simulink model "Copy_of_VTOLTiltrotor"  (R2024a)
settings: configuration reference "VTOLConfiguration" (kept outside this file)
undefined symbols (not defined in the file): airspeed, Battery, BCE12, BCE_Set_init, BMS_Controller_State, C, Cell10_P, Cell11_P, Cell12_P, Cell1_N, Cell1_P, Cell2_P, Cell3_P, Cell4_P, Cell5_P, Cell6_P, Cell7_P, Cell8_P, Cell9_P, Cell_Temperatures, Cell_Voltages, Charging_State, CityMission, control, controlParams, ControlSampleTime, CriticalTiltAngle, currentFactor, CV_Gain, ddx, ddy, ddz, Device_01, DiscIntNeverNeededParam, dx, dy, dz, Earth, env, F, F28379D_ADC_MaxCount, F28379D_ADC_Vmax, FixedWingMission, flightState, Foc_Ki_IxTcpu, Foc_Ki_S, Foc_Kp_I, Foc_Kp_S, fractalcoef, FSState, FWControlParams, HoverMission, I_cc, Ia_offset, Ib_offset, iniRoll, initPitch, iniYaw, IO334, IO334_DAC_Vmax ... (+55)
libraries: slrealtimeethercatlib x109, simulink x81, fl_lib x65, slpidlib x49, mcbcontrolslib x48, nesl_utility x43, speedgoatlib_hdlCoder_IO3xx x31, canmsglib x17, slrealtimeutilitieslib x13, mcbhdlplantlib x13, speedgoatlib_IO611 x12, dspstat3 x12
(part 9 of 20)

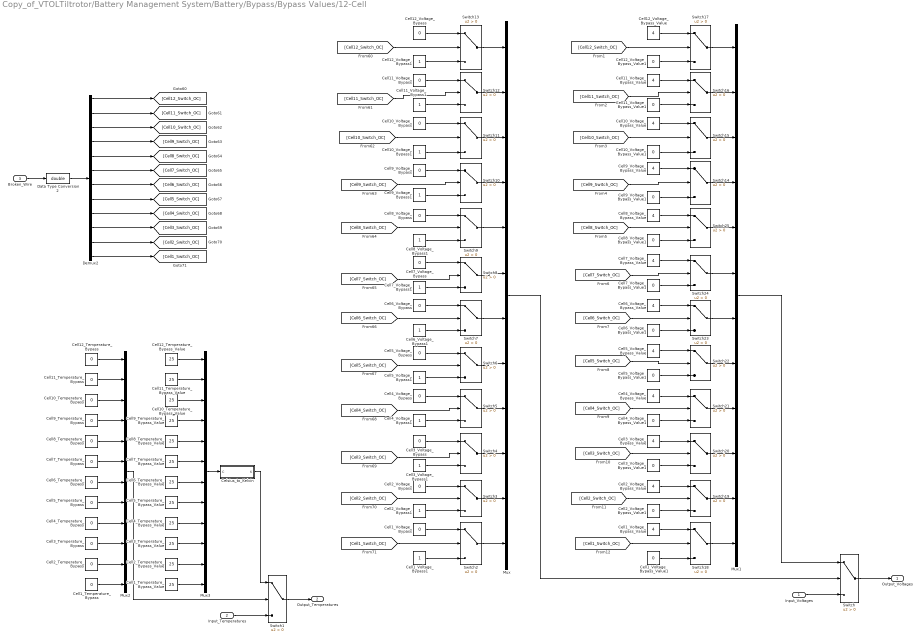
== system Copy_of_VTOLTiltrotor/Battery Management System/Battery/Bypass/Bypass Values/12-Cell ==
  Input_Voltages : Inport
  Input_Temperatures : Inport  Port=2
  Broken_Wire : Inport  Port=3
  Cell10_Temperature_Bypass : Constant  Value=0  SampleTime=-1
  Cell10_Temperature_Bypass_Value : Constant  Value=25  SampleTime=-1
  Cell10_Voltage_Bypass : Constant  Value=0  SampleTime=-1
  Cell10_Voltage_Bypass1 : Constant  SampleTime=-1
  Cell10_Voltage_Bypass_Value : Constant  Value=4  SampleTime=-1
  Cell10_Voltage_Bypass_Value1 : Constant  Value=0  SampleTime=-1
  Cell11_Temperature_Bypass : Constant  Value=0  SampleTime=-1
  Cell11_Temperature_Bypass_Value : Constant  Value=25  SampleTime=-1
  Cell11_Voltage_Bypass : Constant  Value=0  SampleTime=-1
  Cell11_Voltage_Bypass1 : Constant  SampleTime=-1
  Cell11_Voltage_Bypass_Value : Constant  Value=4  SampleTime=-1
  Cell11_Voltage_Bypass_Value1 : Constant  Value=0  SampleTime=-1
  Cell12_Temperature_Bypass : Constant  Value=0  SampleTime=-1
  Cell12_Temperature_Bypass_Value : Constant  Value=25  SampleTime=-1
  Cell12_Voltage_Bypass : Constant  Value=0  SampleTime=-1
  Cell12_Voltage_Bypass1 : Constant  SampleTime=-1
  Cell12_Voltage_Bypass_Value : Constant  Value=4  SampleTime=-1
  Cell12_Voltage_Bypass_Value1 : Constant  Value=0  SampleTime=-1
  Cell1_Temperature_Bypass : Constant  Value=0  SampleTime=-1
  Cell1_Temperature_Bypass_Value : Constant  Value=25  SampleTime=-1
  Cell1_Voltage_Bypass : Constant  Value=0  SampleTime=-1
  Cell1_Voltage_Bypass1 : Constant  SampleTime=-1
  Cell1_Voltage_Bypass_Value : Constant  Value=4  SampleTime=-1
  Cell1_Voltage_Bypass_Value1 : Constant  Value=0  SampleTime=-1
  Cell2_Temperature_Bypass : Constant  Value=0  SampleTime=-1
  Cell2_Temperature_Bypass_Value : Constant  Value=25  SampleTime=-1
  Cell2_Voltage_Bypass : Constant  Value=0  SampleTime=-1
  Cell2_Voltage_Bypass1 : Constant  SampleTime=-1
  Cell2_Voltage_Bypass_Value : Constant  Value=4  SampleTime=-1
  Cell2_Voltage_Bypass_Value1 : Constant  Value=0  SampleTime=-1
  Cell3_Temperature_Bypass : Constant  Value=0  SampleTime=-1
  Cell3_Temperature_Bypass_Value : Constant  Value=25  SampleTime=-1
  Cell3_Voltage_Bypass : Constant  Value=0  SampleTime=-1
  Cell3_Voltage_Bypass1 : Constant  SampleTime=-1
  Cell3_Voltage_Bypass_Value : Constant  Value=4  SampleTime=-1
  Cell3_Voltage_Bypass_Value1 : Constant  Value=0  SampleTime=-1
  Cell4_Temperature_Bypass : Constant  Value=0  SampleTime=-1
  Cell4_Temperature_Bypass_Value : Constant  Value=25  SampleTime=-1
  Cell4_Voltage_Bypass : Constant  Value=0  SampleTime=-1
  Cell4_Voltage_Bypass1 : Constant  SampleTime=-1
  Cell4_Voltage_Bypass_Value : Constant  Value=4  SampleTime=-1
  Cell4_Voltage_Bypass_Value1 : Constant  Value=0  SampleTime=-1
  Cell5_Temperature_Bypass : Constant  Value=0  SampleTime=-1
  Cell5_Temperature_Bypass_Value : Constant  Value=25  SampleTime=-1
  Cell5_Voltage_Bypass : Constant  Value=0  SampleTime=-1
  Cell5_Voltage_Bypass1 : Constant  SampleTime=-1
  Cell5_Voltage_Bypass_Value : Constant  Value=4  SampleTime=-1
  Cell5_Voltage_Bypass_Value1 : Constant  Value=0  SampleTime=-1
  Cell6_Temperature_Bypass : Constant  Value=0  SampleTime=-1
  Cell6_Temperature_Bypass_Value : Constant  Value=25  SampleTime=-1
  Cell6_Voltage_Bypass : Constant  Value=0  SampleTime=-1
  Cell6_Voltage_Bypass1 : Constant  SampleTime=-1
  Cell6_Voltage_Bypass_Value : Constant  Value=4  SampleTime=-1
  Cell6_Voltage_Bypass_Value1 : Constant  Value=0  SampleTime=-1
  Cell7_Temperature_Bypass : Constant  Value=0  SampleTime=-1
  Cell7_Temperature_Bypass_Value : Constant  Value=25  SampleTime=-1
  Cell7_Voltage_Bypass : Constant  Value=0  SampleTime=-1
  Cell7_Voltage_Bypass1 : Constant  SampleTime=-1
  Cell7_Voltage_Bypass_Value : Constant  Value=4  SampleTime=-1
  Cell7_Voltage_Bypass_Value1 : Constant  Value=0  SampleTime=-1
  Cell8_Temperature_Bypass : Constant  Value=0  SampleTime=-1
  Cell8_Temperature_Bypass_Value : Constant  Value=25  SampleTime=-1
  Cell8_Voltage_Bypass : Constant  Value=0  SampleTime=-1
  Cell8_Voltage_Bypass1 : Constant  SampleTime=-1
  Cell8_Voltage_Bypass_Value : Constant  Value=4  SampleTime=-1
  Cell8_Voltage_Bypass_Value1 : Constant  Value=0  SampleTime=-1
  Cell9_Temperature_Bypass : Constant  Value=0  SampleTime=-1
  Cell9_Temperature_Bypass_Value : Constant  Value=25  SampleTime=-1
  Cell9_Voltage_Bypass : Constant  Value=0  SampleTime=-1
  Cell9_Voltage_Bypass1 : Constant  SampleTime=-1
  Cell9_Voltage_Bypass_Value : Constant  Value=4  SampleTime=-1
  Cell9_Voltage_Bypass_Value1 : Constant  Value=0  SampleTime=-1
  Celsius_to_Kelvin : Subsystem
  Data Type Conversion2 : DataTypeConversion  OutDataTypeStr=double  SaturateOnIntegerOverflow=off  RndMeth=Floor
  Demux2 : Demux  Outputs=12
  Mux{,1..3} (4 alike) : Mux  Inputs=12
  Switch{,1..25} (26 alike) : Switch  Criteria=u2 > Threshold  SaturateOnIntegerOverflow=off  InputSameDT=off
  Output_Voltages : Outport
  Output_Temperatures : Outport  Port=2
  wires:
  Mux/1 -> Switch/2
  Switch/1 -> Output_Voltages/1
  Mux1/1 -> Switch/1
  Input_Voltages/1 -> Switch/3
  Cell11_Temperature_Bypass/1 -> Mux2/2
  Cell1_Temperature_Bypass/1 -> Mux2/12
  Cell5_Temperature_Bypass/1 -> Mux2/8
  Cell6_Temperature_Bypass/1 -> Mux2/7
  Cell10_Temperature_Bypass/1 -> Mux2/3
  Cell4_Temperature_Bypass/1 -> Mux2/9
  Cell2_Temperature_Bypass/1 -> Mux2/11
  Cell9_Temperature_Bypass/1 -> Mux2/4
  Cell8_Temperature_Bypass_Value/1 -> Mux3/5
  Cell10_Temperature_Bypass_Value/1 -> Mux3/3
  Mux3/1 -> Celsius_to_Kelvin/1(C)
  Cell12_Temperature_Bypass_Value/1 -> Mux3/1
  Cell1_Temperature_Bypass_Value/1 -> Mux3/12
  Cell11_Temperature_Bypass_Value/1 -> Mux3/2
  Cell8_Temperature_Bypass/1 -> Mux2/5
  Cell3_Temperature_Bypass_Value/1 -> Mux3/10
  Cell9_Temperature_Bypass_Value/1 -> Mux3/4
  Cell6_Temperature_Bypass_Value/1 -> Mux3/7
  Cell12_Temperature_Bypass/1 -> Mux2/1
  Cell5_Temperature_Bypass_Value/1 -> Mux3/8
  Cell2_Temperature_Bypass_Value/1 -> Mux3/11
  Cell7_Temperature_Bypass/1 -> Mux2/6
  Mux2/1 -> Switch1/2
  Celsius_to_Kelvin/1(K) -> Switch1/1
  Cell4_Temperature_Bypass_Value/1 -> Mux3/9
  Input_Temperatures/1 -> Switch1/3
  Cell3_Temperature_Bypass/1 -> Mux2/10
  Cell7_Temperature_Bypass_Value/1 -> Mux3/6
  Switch1/1 -> Output_Temperatures/1
  Switch2/1 -> Mux/12
  [Cell5_Switch_OC] -> Switch6/2
  [Cell1_Switch_OC] -> Switch2/2
  [Cell8_Switch_OC] -> Switch9/2
  [Cell6_Switch_OC] -> Switch7/2
  [Cell7_Switch_OC] -> Switch8/2
  [Cell10_Switch_OC] -> Switch11/2
  [Cell12_Switch_OC] -> Switch13/2
  [Cell3_Switch_OC] -> Switch4/2
  [Cell9_Switch_OC] -> Switch10/2
  [Cell4_Switch_OC] -> Switch5/2
  [Cell11_Switch_OC] -> Switch12/2
  [Cell2_Switch_OC] -> Switch3/2
  Switch3/1 -> Mux/11
  Switch13/1 -> Mux/1
  Switch12/1 -> Mux/2
  Switch11/1 -> Mux/3
  Switch10/1 -> Mux/4
  Switch9/1 -> Mux/5
  Switch8/1 -> Mux/6
  Switch7/1 -> Mux/7
  Switch6/1 -> Mux/8
  Switch5/1 -> Mux/9
  Switch4/1 -> Mux/10
  Cell1_Voltage_Bypass/1 -> Switch2/1
  Cell2_Voltage_Bypass/1 -> Switch3/1
  Cell12_Voltage_Bypass/1 -> Switch13/1
  Cell11_Voltage_Bypass/1 -> Switch12/1
  Cell10_Voltage_Bypass/1 -> Switch11/1
  Cell9_Voltage_Bypass/1 -> Switch10/1
  Cell8_Voltage_Bypass/1 -> Switch9/1
  Cell7_Voltage_Bypass/1 -> Switch8/1
  Cell6_Voltage_Bypass/1 -> Switch7/1
  Cell5_Voltage_Bypass/1 -> Switch6/1
  Cell4_Voltage_Bypass/1 -> Switch5/1
  Cell3_Voltage_Bypass/1 -> Switch4/1
  Cell1_Voltage_Bypass1/1 -> Switch2/3
  Cell2_Voltage_Bypass1/1 -> Switch3/3
  Cell3_Voltage_Bypass1/1 -> Switch4/3
  Cell4_Voltage_Bypass1/1 -> Switch5/3
  Cell5_Voltage_Bypass1/1 -> Switch6/3
  Cell6_Voltage_Bypass1/1 -> Switch7/3
  Cell7_Voltage_Bypass1/1 -> Switch8/3
  Cell8_Voltage_Bypass1/1 -> Switch9/3
  Cell9_Voltage_Bypass1/1 -> Switch10/3
  Cell10_Voltage_Bypass1/1 -> Switch11/3
  Cell11_Voltage_Bypass1/1 -> Switch12/3
  Cell12_Voltage_Bypass1/1 -> Switch13/3
  Switch17/1 -> Mux1/1
  Switch16/1 -> Mux1/2
  Switch18/1 -> Mux1/12
  Switch25/1 -> Mux1/5
  Switch20/1 -> Mux1/10
  Switch19/1 -> Mux1/11
  Switch15/1 -> Mux1/3
  Switch14/1 -> Mux1/4
  Switch24/1 -> Mux1/6
  Switch23/1 -> Mux1/7
  Switch22/1 -> Mux1/8
  Switch21/1 -> Mux1/9
  Cell12_Voltage_Bypass_Value/1 -> Switch17/1
  Cell11_Voltage_Bypass_Value/1 -> Switch16/1
  Cell10_Voltage_Bypass_Value/1 -> Switch15/1
  Cell9_Voltage_Bypass_Value/1 -> Switch14/1
  Cell8_Voltage_Bypass_Value/1 -> Switch25/1
  Cell6_Voltage_Bypass_Value/1 -> Switch23/1
  Cell5_Voltage_Bypass_Value/1 -> Switch22/1
  Cell4_Voltage_Bypass_Value/1 -> Switch21/1
  Cell3_Voltage_Bypass_Value/1 -> Switch20/1
  Cell2_Voltage_Bypass_Value/1 -> Switch19/1
  Cell1_Voltage_Bypass_Value/1 -> Switch18/1
  Cell7_Voltage_Bypass_Value/1 -> Switch24/1
  Cell12_Voltage_Bypass_Value1/1 -> Switch17/3
  Cell11_Voltage_Bypass_Value1/1 -> Switch16/3
  Cell10_Voltage_Bypass_Value1/1 -> Switch15/3
  Cell9_Voltage_Bypass_Value1/1 -> Switch14/3
  Cell8_Voltage_Bypass_Value1/1 -> Switch25/3
  Cell7_Voltage_Bypass_Value1/1 -> Switch24/3
  Cell6_Voltage_Bypass_Value1/1 -> Switch23/3
  Cell5_Voltage_Bypass_Value1/1 -> Switch22/3
  Cell4_Voltage_Bypass_Value1/1 -> Switch21/3
  Cell3_Voltage_Bypass_Value1/1 -> Switch20/3
  Cell2_Voltage_Bypass_Value1/1 -> Switch19/3
  Cell1_Voltage_Bypass_Value1/1 -> Switch18/3
  [Cell12_Switch_OC] -> Switch17/2
  [Cell10_Switch_OC] -> Switch15/2
  [Cell11_Switch_OC] -> Switch16/2
  [Cell9_Switch_OC] -> Switch14/2
  [Cell8_Switch_OC] -> Switch25/2
  [Cell7_Switch_OC] -> Switch24/2
  [Cell6_Switch_OC] -> Switch23/2
  [Cell5_Switch_OC] -> Switch22/2
  [Cell4_Switch_OC] -> Switch21/2
  [Cell3_Switch_OC] -> Switch20/2
  [Cell2_Switch_OC] -> Switch19/2
  [Cell1_Switch_OC] -> Switch18/2
  Demux2/6 -> [Cell7_Switch_OC]
  Demux2/12 -> [Cell1_Switch_OC]
  Broken_Wire/1 -> Data Type Conversion2/1
  Demux2/5 -> [Cell8_Switch_OC]
  Demux2/11 -> [Cell2_Switch_OC]
  Demux2/7 -> [Cell6_Switch_OC]
  Demux2/3 -> [Cell10_Switch_OC]
  Demux2/9 -> [Cell4_Switch_OC]
  Demux2/2 -> [Cell11_Switch_OC]
  Demux2/10 -> [Cell3_Switch_OC]
  Demux2/4 -> [Cell9_Switch_OC]
  Demux2/8 -> [Cell5_Switch_OC]
  Data Type Conversion2/1 -> Demux2/1
  Demux2/1 -> [Cell12_Switch_OC]

== system Copy_of_VTOLTiltrotor/Battery Management System/Battery/HW Interface/BCE - HIL/Battery Cell Emulator ==
  Sensor_Values_Sim : Inport
  "BCE Bus Packing " : Subsystem
  "BCE Read " : Subsystem  InitFcn=sg_bce.checkNumberOfBlocksGlobal(bdroot);  mask(bce_read){}
      settings: OpenFcn=sg_bce.openFcnRead;
      mask Help: eval('sg.utils.help.show(''io_main/refentry_bce_read'');')
      mask Display: disp('Speedgoat\nBMTS Read\nEtherCAT Bus: 0, Device: 1\nBCE12-0505');port_label('output',1,'Data');
  "BCE Setup " : Subsystem  LoadFcn=|  InitFcn=|  mask(bce_setup){}
      LoadFcn=|
      | sg_bce.createBusSignals;
      | sg_bce.setupEniCallback(gcb, bdroot);
      InitFcn=|
      | sg_bce.createBusSignals;
      | sg_bce.checkNumberOfBlocksGlobal(bdroot);
      | sg_bce.setupEniCallback(gcb, bdroot);
      settings: OpenFcn=sg_bce.openFcnSetup;
      mask Help: eval('sg.utils.help.show(''io_main/refentry_bce_setup'');')
      mask Display: disp('Speedgoat\nBattery Management Testing Systems\nEtherCAT Bus: 0\nSetup');
  "BCE Write " : Subsystem  InitFcn=sg_bce.checkNumberOfBlocksGlobal(bdroot);  mask(bce_write){}
      settings: OpenFcn=sg_bce.openFcnWrite;
      mask Help: eval('sg.utils.help.show(''io_main/refentry_bce_write'');')
      mask Display: disp('Speedgoat\nBMTS Write\nEtherCAT Bus: 0, Device: 1\nBCE12-0505');port_label('input',1,'Data');
  BCE_Init : Switch  Criteria=u2 > Threshold  SaturateOnIntegerOverflow=off  InputSameDT=off
  Bus Selector : BusSelector  OutputSignals=Cell_12.I,Cell_11.I,Cell_10.I,Cell_9.I,Cell_8.I,Cell_7.I,Cell_6.I,Cell_5.I,Cell_4.I,Cell_3.I,Cell_2.I,Cell_1.I
  Bus Selector1 : BusSelector  OutputSignals=Cell_Voltages
  Bus Selector2 : BusSelector  OutputSignals=Cell_12.V,Cell_11.V,Cell_10.V,Cell_9.V,Cell_8.V,Cell_7.V,Cell_6.V,Cell_5.V,Cell_4.V,Cell_3.V,Cell_2.V,Cell_1.V
  Constant : Constant  Value=[0,0,0,0,0,0,0,0,0,0,0,0]
  Data Type Conversion : DataTypeConversion  OutDataTypeStr=single  SaturateOnIntegerOverflow=off  RndMeth=Floor
  Data Type Conversion1 : DataTypeConversion  OutDataTypeStr=boolean  SaturateOnIntegerOverflow=off  RndMeth=Floor
  Data Type Conversion2 : DataTypeConversion  OutDataTypeStr=single  SaturateOnIntegerOverflow=off  RndMeth=Floor
  Demux : Demux  Outputs=12
  Enable : Constant
  Mux : Mux  Inputs=12
  Mux1 : Mux  Inputs=12
  No_current : Constant  Value=0
  Step : Step  Time=2
  Current_Values : Outport
  Cell_Voltages : Outport  Port=2
  wires:
  Sensor_Values_Sim/1 -> Bus Selector1/1
  BCE_Init/1 -> Demux/1
  "BCE Read "/1(Data) -> Bus Selector/1, Bus Selector2/1
  Constant/1 -> Data Type Conversion2/1
  Step/1 -> BCE_Init/2
  "BCE Bus Packing "/1(BCE Bus) -> "BCE Write "/1(Data)
  No_current/1 -> Data Type Conversion/1
  Data Type Conversion2/1 -> BCE_Init/3
  Bus Selector/1 -> Mux/1  "<I>"
  Bus Selector/2 -> Mux/2  "<I>"
  Bus Selector/3 -> Mux/3  "<I>"
  Bus Selector/4 -> Mux/4  "<I>"
  Bus Selector/5 -> Mux/5  "<I>"
  Bus Selector/6 -> Mux/6  "<I>"
  Bus Selector/7 -> Mux/7  "<I>"
  Bus Selector/8 -> Mux/8  "<I>"
  Bus Selector/9 -> Mux/9  "<I>"
  Bus Selector/10 -> Mux/10  "<I>"
  Bus Selector/11 -> Mux/11  "<I>"
  Bus Selector/12 -> Mux/12  "<I>"
  Mux/1 -> Current_Values/1
  Bus Selector2/1 -> Mux1/1  "<V>"
  Bus Selector2/2 -> Mux1/2  "<V>"
  Bus Selector2/3 -> Mux1/3  "<V>"
  Bus Selector2/4 -> Mux1/4  "<V>"
  Bus Selector2/5 -> Mux1/5  "<V>"
  Bus Selector2/6 -> Mux1/6  "<V>"
  Bus Selector2/7 -> Mux1/7  "<V>"
  Bus Selector2/8 -> Mux1/8  "<V>"
  Bus Selector2/9 -> Mux1/9  "<V>"
  Bus Selector2/10 -> Mux1/10  "<V>"
  Bus Selector2/11 -> Mux1/11  "<V>"
  Bus Selector2/12 -> Mux1/12  "<V>"
  Mux1/1 -> Cell_Voltages/1
  Bus Selector1/1 -> BCE_Init/1  "<Cell_Voltages>"
  Enable/1 -> Data Type Conversion1/1
  Data Type Conversion1/1 -> "BCE Bus Packing "/1(Cell 1 Enable), "BCE Bus Packing "/9(Cell 9 Enable), "BCE Bus Packing "/12(Cell 12 Enable), "BCE Bus Packing "/11(Cell 11 Enable), "BCE Bus Packing "/10(Cell 10 Enable), "BCE Bus Packing "/8(Cell 8 Enable), "BCE Bus Packing "/7(Cell 7 Enable), "BCE Bus Packing "/6(Cell 6 Enable), "BCE Bus Packing "/5(Cell 5 Enable), "BCE Bus Packing "/4(Cell 4 Enable), "BCE Bus Packing "/3(Cell 3 Enable), "BCE Bus Packing "/2(Cell 2 Enable)
  Data Type Conversion/1 -> "BCE Bus Packing "/29(Cell 5 Current), "BCE Bus Packing "/28(Cell 4 Current), "BCE Bus Packing "/25(Cell 1 Current), "BCE Bus Packing "/26(Cell 2 Current), "BCE Bus Packing "/27(Cell 3 Current), "BCE Bus Packing "/30(Cell 6 Current), "BCE Bus Packing "/31(Cell 7 Current), "BCE Bus Packing "/32(Cell 8 Current), "BCE Bus Packing "/33(Cell 9 Current), "BCE Bus Packing "/34(Cell 10 Current), "BCE Bus Packing "/35(Cell 11 Current), "BCE Bus Packing "/36(Cell 12 Current)
  Demux/1 -> "BCE Bus Packing "/13(Cell 12 Voltage)
  Demux/2 -> "BCE Bus Packing "/14(Cell 11 Voltage)
  Demux/3 -> "BCE Bus Packing "/15(Cell 10 Voltage)
  Demux/4 -> "BCE Bus Packing "/16(Cell 9 Voltage)
  Demux/5 -> "BCE Bus Packing "/17(Cell 8 Voltage)
  Demux/6 -> "BCE Bus Packing "/18(Cell 7 Voltage)
  Demux/7 -> "BCE Bus Packing "/19(Cell 6 Voltage)
  Demux/8 -> "BCE Bus Packing "/20(Cell 5 Voltage)
  Demux/9 -> "BCE Bus Packing "/21(Cell 4 Voltage)
  Demux/10 -> "BCE Bus Packing "/22(Cell 3 Voltage)
  Demux/11 -> "BCE Bus Packing "/23(Cell 2 Voltage)
  Demux/12 -> "BCE Bus Packing "/24(Cell 1 Voltage)

== system Copy_of_VTOLTiltrotor/Battery Management System/Battery/HW Interface/BCE - HIL/Shunt Emulator ==
  note: Shunt Emulator Blocks
  Sensor_Values_Sim : Inport
  Bus Selector : BusSelector  OutputSignals=Pack_Current
  Pack_Current : Outport
  wires:
  Sensor_Values_Sim/1 -> Bus Selector/1
  Bus Selector/1 -> Pack_Current/1  "<Pack_Current>"

== system Copy_of_VTOLTiltrotor/Battery Management System/Battery/HW Interface/BCE - HIL/Temperature Emulator ==
  note: Temperature Emulation Blocks
  Sensor_Values_Sim : Inport
  Bus Selector : BusSelector  OutputSignals=Cell_Temperatures
  Cell_Temperatures : Outport
  wires:
  Sensor_Values_Sim/1 -> Bus Selector/1
  Bus Selector/1 -> Cell_Temperatures/1  "<Cell_Temperatures>"

== system Copy_of_VTOLTiltrotor/Battery Management System/Instrumentation/Instrumented Signals/12-Cell/Celsius_to_Kelvin ==
  K : Inport
  Add : Sum  Inputs=+-
  Constant4 : Constant  Value=273.15
  C : Outport
  wires:
  Constant4/1 -> Add/2
  K/1 -> Add/1
  Add/1 -> C/1

== system Copy_of_VTOLTiltrotor/Dynamics/Force and Moments/Aerodynamic Forces/Compute Body Frame Forces and Moments/Rotate FM to body frame ==
  FM_w : Inport
  alpha_beta : Inport  Port=2
  Forces : Selector  InputPortWidth=6  IndexOptions=Index vector (dialog)  Indices=[1 2 3]  OutputSizes=[(-2)]
  Moments : Selector  InputPortWidth=6  IndexOptions=Index vector (dialog)  Indices=[4 5 6]  OutputSizes=[(-2)]
  Rotate Forces : Subsystem
  Rotate Moments : Subsystem
  F_b : Outport  VectorParamsAs1DForOutWhenUnconnected=off
  M_b : Outport  Port=2  VectorParamsAs1DForOutWhenUnconnected=off
  wires:
  alpha_beta/1 -> Rotate Forces/2(alpha_beta), Rotate Moments/1(alpha_beta)
  Moments/1 -> Rotate Moments/2(M_w)
  FM_w/1 -> Moments/1, Forces/1
  Forces/1 -> Rotate Forces/1(F_w)
  Rotate Moments/1(M_b) -> M_b/1
  Rotate Forces/1(F_b) -> F_b/1

== system Copy_of_VTOLTiltrotor/Dynamics/Force and Moments/Aerodynamic Forces/Compute Body Frame Forces and Moments/Wind frame F& M ==
  Airdata : Inport
  CtrlSurfaces : Inport  Port=2
  p,q,r : Inport  Port=3
  Bus Creator1 : BusCreator  Inputs=2
  Bus Selector1 : BusSelector  OutputSignals=dA,dR
  Bus Selector2 : BusSelector  OutputSignals=dE,dA,dR
  Bus Selector6 : BusSelector  OutputSignals=beta,airspeed
  Bus Selector7 : BusSelector  OutputSignals=alpha,airspeed
  Get Forces and Moments : Subsystem
  Lateral Channel : Subsystem
  Longitudinal Channel : Subsystem
  FM_w : Outport  PortDimensions=6  VectorParamsAs1DForOutWhenUnconnected=off
  wires:
  Get Forces and Moments/1(FM_w) -> FM_w/1
  Bus Creator1/1 -> Get Forces and Moments/2(AeroCoeffs)
  Bus Selector7/2 -> Longitudinal Channel/2(Airpseed)  "<airspeed>"
  Bus Selector7/1 -> Longitudinal Channel/1(alpha)  "<alpha>"
  Bus Selector6/2 -> Lateral Channel/2(Airspeed)  "<airspeed>"
  Bus Selector6/1 -> Lateral Channel/1(beta)  "<beta>"
  Airdata/1 -> Bus Selector6/1, Bus Selector7/1, Get Forces and Moments/1(Airdata)
  Bus Selector2/1 -> Longitudinal Channel/3(dE)  "<dE>"
  Bus Selector1/2 -> Lateral Channel/4(dR)  "<dR>"
  Bus Selector1/1 -> Lateral Channel/3(dA)  "<dA>"
  CtrlSurfaces/1 -> Bus Selector1/1, Bus Selector2/1
  p,q,r/1 -> Lateral Channel/5(p,q,r), Longitudinal Channel/4(p,q,r)
  Lateral Channel/1(Lateral) -> Bus Creator1/1
  Longitudinal Channel/1(Longitudinal) -> Bus Creator1/2
  Bus Selector2/2 -> Longitudinal Channel/5(dA)  "<dA>"
  Bus Selector2/3 -> Longitudinal Channel/6(dR)  "<dR>"

== system Copy_of_VTOLTiltrotor/Flight Controller/Autopilot/Fixed Wing Controller/Fixed Wing Controller Simulation/AER from Path Manager ==
  In1 : Inport
  Enable : EnablePort
  Out1 : Outport
  wires:
  In1/1 -> Out1/1

== system Copy_of_VTOLTiltrotor/Flight Controller/Autopilot/Fixed Wing Controller/Fixed Wing Controller Simulation/Airspeed-Altitude Controller ==
  note: Airspeed and altitude are controlled independently
      | by ignoring their coupled dynamics.
  Airspeed SP : Inport
  Altitude SP : Inport  Port=2
  Climb Rate SP : Inport  Port=3
  Airspeed : Inport  Port=4
  xyz : Inport  Port=5
  vxyz : Inport  Port=6
  Enable : EnablePort  ShowOutputPort=on
  Airspeed Controller : slpidlib/PID Controller  Controller=PID  Form=Parallel  TimeDomain=Discrete-time  UseExternalTs=off  SampleTime=ControlSampleTime  IntegratorMethod=Trapezoidal  FilterMethod=Forward Euler  ControllerParametersSource=internal  P=FWControlParams.P_AIRSPD  I=FWControlParams.I_AIRSPD  UseKiTs=off  D=FWControlParams.D_AIRSPD  UseExternalDerivativeSource=off  N=FWControlParams.N_AIRSPD  UseFilter=on  TunerSelectOption=Transfer Function Based (PID Tuner App)  InitialConditionSource=internal  InitialConditionForIntegrator=0  InitialConditionForFilter=0  DifferentiatorICPrevScaledInput=0  ExternalReset=none  TrackingMode=off  Kt=1  LimitOutput=off  SatLimitsSource=internal  UpperSaturationLimit=Inf  LowerSaturationLimit=0  LinearizeAsGain=on  AntiWindupMode=clamping  Kb=1  LimitIntegrator=off  UpperIntegratorSaturationLimit=inf  LowerIntegratorSaturationLimit=-inf  POutMin=[]  POutMax=[]  IOutMin=[]  IOutMax=[]  DOutMin=[]  DOutMax=[]  NOutMin=[]  NOutMax=[]  SumOutMin=[]  SumOutMax=[]  SaturationOutMin=[]  SaturationOutMax=[]  PParamMin=[]  PParamMax=[]  IParamMin=[]  IParamMax=[]  DParamMin=[]  DParamMax=[]  NParamMin=[]  NParamMax=[]  KbParamMin=[]  KbParamMax=[]  KtParamMin=[]  KtParamMax=[]  KbOutMin=[]  KbOutMax=[]  KtOutMin=[]  KtOutMax=[]  IntegratorOutMin=[]  IntegratorOutMax=[]  FilterOutMin=[]  FilterOutMax=[]  SumI1OutMin=[]  SumI1OutMax=[]  SumI2OutMin=[]  SumI2OutMax=[]  SumI3OutMin=[]  SumI3OutMax=[]  SumI4OutMin=[]  SumI4OutMax=[]  SumDOutMin=[]  SumDOutMax=[]  DifferentiatorOutMin=[]  DifferentiatorOutMax=[]  FilterDiffOutCoefMin=[]  FilterDiffOutCoefMax=[]  ReciprocalOutMin=[]  ReciprocalOutMax=[]  SumDenOutMin=[]  SumDenOutMax=[]  SumNumOutMin=[]  SumNumOutMax=[]  DivideOutMin=[]  DivideOutMax=[]  UdiffTsProdOutMin=[]  UdiffTsProdOutMax=[]  NTsProdOutMin=[]  NTsProdOutMax=[]  UintegralTsProdOutMin=[]  UintegralTsProdOutMax=[]  UngainTsProdOutMin=[]  UngainTsProdOutMax=[]  ClampingZeroOutDataTypeStr=Inherit: Inherit via back propagation  ClampingZeroOutMin=[]  ClampingZeroOutMax=[]  FilterDenConstantOutDataTypeStr=Inherit: Inherit via back propagation  FilterDenConstantOutMin=[]  FilterDenConstantOutMax=[]  PCopyOutDataTypeStr=Inherit: Inherit via back propagation  PCopyOutMin=[]  PCopyOutMax=[]  NCopyOutDataTypeStr=Inherit: Inherit via back propagation  NCopyOutMin=[]  NCopyOutMax=[]  IntegratorContinuousStateAttributes=''  IntegratorStateMustResolveToSignalObject=off  IntegratorRTWStateStorageClass=Auto  FilterContinuousStateAttributes=''  FilterStateMustResolveToSignalObject=off  FilterRTWStateStorageClass=Auto  ParallelPVariant=InternalParameters  IdealPVariant=Disabled  IVariant=InternalParameters  DVariant=InternalParameters  IntegratorVariant=Discrete  SatVariant=Disabled  AWVariant=Passthrough  PCopyVariant=Disabled  TRVariant=Disabled  FdbkBlocksVariant=Forward  IdealPFdbkVariant=Disabled  SatFdbkVariant=Disabled  DerivativeFilterVariant=ForwardEulerFilter  NVariant=InternalParameters  NCopyVariant=Disabled  FilterICVariant=InternalICsFilter  IntegratorICVariant=InternalICs  ExternalResetVariant=Disabled  TRSumVariant=Passthrough  SumFdbkVariant=Disabled  SumVariant=Sum_PID  TsampFilterVariant=InternalTs  TsampNgainVariant=Passthrough  TsampIntegralVariant=Disabled_SignalSpec  ExternalSaturationOutDataTypeStr=Inherit: Same as second input  DerivativeSourceVariant=ErrorSignal
  Altitude controller : Subsystem
  Climb Rate SP Merge : Merge
  Climb Rate SP from Guidance : Subsystem  TreatAsAtomicUnit=on
  Compare To Constant : simulink/Logic and Bit Operations/Compare To Constant  relop===  const=uint8(1)  OutDataTypeStr=boolean
  Compare To Constant1 : simulink/Logic and Bit Operations/Compare To Constant  relop===  const=uint8(2)  OutDataTypeStr=boolean
  Pitch SP Controller : Subsystem
  Sum1 : Sum  Inputs=|+-
  Pitch SP : Outport
  Throttle : Outport  Port=2
  wires:
  Airspeed SP/1 -> Sum1/1
  Sum1/1 -> Airspeed Controller/1
  Airspeed/1 -> Sum1/2
  Airspeed Controller/1 -> Throttle/1
  Altitude SP/1 -> Altitude controller/1(Alt SP)
  xyz/1 -> Altitude controller/2(xyz)
  vxyz/1 -> Pitch SP Controller/2(vxyz)
  Pitch SP Controller/1(Pitch SP) -> Pitch SP/1
  Enable/1 -> Compare To Constant1/1, Compare To Constant/1
  Compare To Constant/1 -> Altitude controller/Enable
  Compare To Constant1/1 -> Climb Rate SP from Guidance/Enable
  Altitude controller/1(Climb Rate SP) -> Climb Rate SP Merge/1
  Climb Rate SP from Guidance/1(Out1) -> Climb Rate SP Merge/2
  Climb Rate SP Merge/1 -> Pitch SP Controller/1(Climb Rate SP)
  Climb Rate SP/1 -> Climb Rate SP from Guidance/1(Climb Rate SP)

== system Copy_of_VTOLTiltrotor/Flight Controller/Autopilot/Fixed Wing Controller/Fixed Wing Controller Simulation/Attitude Controller ==
  YPR SP : Inport
  ypr : Inport  Port=2
  Ang Rate : Inport  Port=3
  Airspeed : Inport  Port=4
  Enable : EnablePort  ShowOutputPort=on
  AER Merge : Merge
  Compare To Constant : simulink/Logic and Bit Operations/Compare To Constant  relop===  const=uint8(1)  OutDataTypeStr=boolean
  Compare To Constant1 : simulink/Logic and Bit Operations/Compare To Constant  relop===  const=uint8(2)  OutDataTypeStr=boolean
  Demux1 : Demux  Outputs=3
  Pitch Roll Controller : Subsystem
  Rudder Heading Controller : Subsystem
  AER : Outport
  wires:
  ypr/1 -> Rudder Heading Controller/2(YPR), Pitch Roll Controller/3(YPR)
  YPR SP/1 -> Demux1/1
  Enable/1 -> Compare To Constant1/1, Compare To Constant/1
  AER Merge/1 -> AER/1
  Compare To Constant/1 -> Pitch Roll Controller/Enable
  Pitch Roll Controller/1(AER) -> AER Merge/1
  Rudder Heading Controller/1(AER) -> AER Merge/2
  Demux1/1 -> Rudder Heading Controller/1(Yaw SP)
  Demux1/2 -> Pitch Roll Controller/1(Pitch SP)
  Demux1/3 -> Pitch Roll Controller/2(Roll SP)
  Ang Rate/1 -> Rudder Heading Controller/3(Ang Rate), Pitch Roll Controller/4(Ang Rate)
  Compare To Constant1/1 -> Rudder Heading Controller/Enable
  Airspeed/1 -> Pitch Roll Controller/5(Airspeed)

== system Copy_of_VTOLTiltrotor/Flight Controller/Autopilot/Fixed Wing Controller/Fixed Wing Controller Simulation/Lateral Guidance Logic ==
  note: S. Park, J. Deyst, and J. P. How, "A New Nonlinear Guidance Logic for Trajectory Tracking," Proceedings of the AIAA Guidance, Navigation and Control Conference, Aug 2004. AIAA-2004-4900.
  Course SP : Inport
  L1 Distance : Inport  Port=2
  course : Inport  Port=3
  gndspeed : Inport  Port=4
  Enable : EnablePort
  MATLAB Function : MATLAB Function  TreatAsAtomicUnit=on  SystemSampleTime=ControlSampleTime
  Terminator : Terminator
  Roll SP : Outport
  wires:
  Course SP/1 -> MATLAB Function/1(courseSP)
  course/1 -> MATLAB Function/2(course)
  MATLAB Function/2(rollSP) -> Roll SP/1
  MATLAB Function/1(lacc) -> Terminator/1
  gndspeed/1 -> MATLAB Function/3(groundSpeed)
  L1 Distance/1 -> MATLAB Function/4(L1)

== system Copy_of_VTOLTiltrotor/Flight Controller/Autopilot/Fixed Wing Controller/Fixed Wing Controller Simulation/Pitch, Airspeed SP from Controller ==
  Pitch SP In : Inport
  Airspeed SP : Inport  Port=2
  Airspeed : Inport  Port=3
  Enable : EnablePort
  Airspeed Controller : slpidlib/PID Controller  Controller=PID  Form=Parallel  TimeDomain=Discrete-time  UseExternalTs=off  SampleTime=ControlSampleTime  IntegratorMethod=Trapezoidal  FilterMethod=Forward Euler  ControllerParametersSource=internal  P=FWControlParams.P_AIRSPD  I=FWControlParams.I_AIRSPD  UseKiTs=off  D=FWControlParams.D_AIRSPD  UseExternalDerivativeSource=off  N=FWControlParams.N_AIRSPD  UseFilter=on  TunerSelectOption=Transfer Function Based (PID Tuner App)  InitialConditionSource=internal  InitialConditionForIntegrator=0  InitialConditionForFilter=0  DifferentiatorICPrevScaledInput=0  ExternalReset=none  TrackingMode=off  Kt=1  LimitOutput=off  SatLimitsSource=internal  UpperSaturationLimit=Inf  LowerSaturationLimit=0  LinearizeAsGain=on  AntiWindupMode=clamping  Kb=1  LimitIntegrator=off  UpperIntegratorSaturationLimit=inf  LowerIntegratorSaturationLimit=-inf  POutMin=[]  POutMax=[]  IOutMin=[]  IOutMax=[]  DOutMin=[]  DOutMax=[]  NOutMin=[]  NOutMax=[]  SumOutMin=[]  SumOutMax=[]  SaturationOutMin=[]  SaturationOutMax=[]  PParamMin=[]  PParamMax=[]  IParamMin=[]  IParamMax=[]  DParamMin=[]  DParamMax=[]  NParamMin=[]  NParamMax=[]  KbParamMin=[]  KbParamMax=[]  KtParamMin=[]  KtParamMax=[]  KbOutMin=[]  KbOutMax=[]  KtOutMin=[]  KtOutMax=[]  IntegratorOutMin=[]  IntegratorOutMax=[]  FilterOutMin=[]  FilterOutMax=[]  SumI1OutMin=[]  SumI1OutMax=[]  SumI2OutMin=[]  SumI2OutMax=[]  SumI3OutMin=[]  SumI3OutMax=[]  SumI4OutMin=[]  SumI4OutMax=[]  SumDOutMin=[]  SumDOutMax=[]  DifferentiatorOutMin=[]  DifferentiatorOutMax=[]  FilterDiffOutCoefMin=[]  FilterDiffOutCoefMax=[]  ReciprocalOutMin=[]  ReciprocalOutMax=[]  SumDenOutMin=[]  SumDenOutMax=[]  SumNumOutMin=[]  SumNumOutMax=[]  DivideOutMin=[]  DivideOutMax=[]  UdiffTsProdOutMin=[]  UdiffTsProdOutMax=[]  NTsProdOutMin=[]  NTsProdOutMax=[]  UintegralTsProdOutMin=[]  UintegralTsProdOutMax=[]  UngainTsProdOutMin=[]  UngainTsProdOutMax=[]  ClampingZeroOutDataTypeStr=Inherit: Inherit via back propagation  ClampingZeroOutMin=[]  ClampingZeroOutMax=[]  FilterDenConstantOutDataTypeStr=Inherit: Inherit via back propagation  FilterDenConstantOutMin=[]  FilterDenConstantOutMax=[]  PCopyOutDataTypeStr=Inherit: Inherit via back propagation  PCopyOutMin=[]  PCopyOutMax=[]  NCopyOutDataTypeStr=Inherit: Inherit via back propagation  NCopyOutMin=[]  NCopyOutMax=[]  IntegratorContinuousStateAttributes=''  IntegratorStateMustResolveToSignalObject=off  IntegratorRTWStateStorageClass=Auto  FilterContinuousStateAttributes=''  FilterStateMustResolveToSignalObject=off  FilterRTWStateStorageClass=Auto  ParallelPVariant=InternalParameters  IdealPVariant=Disabled  IVariant=InternalParameters  DVariant=InternalParameters  IntegratorVariant=Discrete  SatVariant=Disabled  AWVariant=Passthrough  PCopyVariant=Disabled  TRVariant=Disabled  FdbkBlocksVariant=Forward  IdealPFdbkVariant=Disabled  SatFdbkVariant=Disabled  DerivativeFilterVariant=ForwardEulerFilter  NVariant=InternalParameters  NCopyVariant=Disabled  FilterICVariant=InternalICsFilter  IntegratorICVariant=InternalICs  ExternalResetVariant=Disabled  TRSumVariant=Passthrough  SumFdbkVariant=Disabled  SumVariant=Sum_PID  TsampFilterVariant=InternalTs  TsampNgainVariant=Passthrough  TsampIntegralVariant=Disabled_SignalSpec  ExternalSaturationOutDataTypeStr=Inherit: Same as second input  DerivativeSourceVariant=ErrorSignal
  IC : InitialCondition  Value=0
  Sum1 : Sum  Inputs=|+-
  Pitch SP : Outport
  Throttle : Outport  Port=2
  wires:
  IC/1 -> Pitch SP/1
  Pitch SP In/1 -> IC/1
  Airspeed SP/1 -> Sum1/1
  Sum1/1 -> Airspeed Controller/1
  Airspeed/1 -> Sum1/2
  Airspeed Controller/1 -> Throttle/1

== system Copy_of_VTOLTiltrotor/Flight Controller/Autopilot/Fixed Wing Controller/Fixed Wing Controller Simulation/Roll SP from Path Manager ==
  In1 : Inport
  Enable : EnablePort
  IC : InitialCondition  Value=0
  Out1 : Outport
  wires:
  In1/1 -> IC/1
  IC/1 -> Out1/1

== system Copy_of_VTOLTiltrotor/Flight Controller/Autopilot/Fixed Wing Controller/Fixed Wing Controller Simulation/Subsystem2 ==
  Euler : Inport
  pqr : Inport  Port=2
  Demux : Demux  Outputs=3
  Display : Display
  MATLAB Function : MATLAB Function  TreatAsAtomicUnit=on
  Matrix Multiply : Product  Multiplication=Matrix(*)
  Terminator : Terminator
  Euler Rate : Outport
  wires:
  Demux/1 -> MATLAB Function/1(phi)
  Demux/2 -> MATLAB Function/2(theta)
  MATLAB Function/1(y) -> Matrix Multiply/1
  pqr/1 -> Matrix Multiply/2
  Euler/1 -> Demux/1
  Demux/3 -> Terminator/1
  Matrix Multiply/1 -> Display/1, Euler Rate/1

== system Copy_of_VTOLTiltrotor/Flight Controller/Autopilot/Fixed Wing Controller/Fixed Wing Controller Tuning/AER from Path Manager ==
  In1 : Inport
  Enable : EnablePort
  Out1 : Outport
  wires:
  In1/1 -> Out1/1

== system Copy_of_VTOLTiltrotor/Flight Controller/Autopilot/Fixed Wing Controller/Fixed Wing Controller Tuning/Airspeed-Altitude Controller ==
  note: Airspeed and altitude are controlled independently
      | by ignoring their coupled dynamics.
  Airspeed SP : Inport
  Altitude SP : Inport  Port=2
  Climb Rate SP : Inport  Port=3
  Airspeed : Inport  Port=4
  xyz : Inport  Port=5
  vxyz : Inport  Port=6
  Enable : EnablePort  ShowOutputPort=on
  Airspeed Controller : slpidlib/PID Controller  Controller=PID  Form=Parallel  TimeDomain=Discrete-time  UseExternalTs=off  SampleTime=ControlSampleTime  IntegratorMethod=Trapezoidal  FilterMethod=Forward Euler  ControllerParametersSource=internal  P=40.1166410885074  I=21.6851560041072  UseKiTs=off  D=2.18528545905044  UseExternalDerivativeSource=off  N=172.44752694034  UseFilter=on  TunerSelectOption=Transfer Function Based (PID Tuner App)  InitialConditionSource=internal  InitialConditionForIntegrator=0  InitialConditionForFilter=0  DifferentiatorICPrevScaledInput=0  ExternalReset=none  TrackingMode=off  Kt=1  LimitOutput=off  SatLimitsSource=internal  UpperSaturationLimit=Inf  LowerSaturationLimit=0  LinearizeAsGain=on  AntiWindupMode=clamping  Kb=1  LimitIntegrator=off  UpperIntegratorSaturationLimit=inf  LowerIntegratorSaturationLimit=-inf  POutMin=[]  POutMax=[]  IOutMin=[]  IOutMax=[]  DOutMin=[]  DOutMax=[]  NOutMin=[]  NOutMax=[]  SumOutMin=[]  SumOutMax=[]  SaturationOutMin=[]  SaturationOutMax=[]  PParamMin=[]  PParamMax=[]  IParamMin=[]  IParamMax=[]  DParamMin=[]  DParamMax=[]  NParamMin=[]  NParamMax=[]  KbParamMin=[]  KbParamMax=[]  KtParamMin=[]  KtParamMax=[]  KbOutMin=[]  KbOutMax=[]  KtOutMin=[]  KtOutMax=[]  IntegratorOutMin=[]  IntegratorOutMax=[]  FilterOutMin=[]  FilterOutMax=[]  SumI1OutMin=[]  SumI1OutMax=[]  SumI2OutMin=[]  SumI2OutMax=[]  SumI3OutMin=[]  SumI3OutMax=[]  SumI4OutMin=[]  SumI4OutMax=[]  SumDOutMin=[]  SumDOutMax=[]  DifferentiatorOutMin=[]  DifferentiatorOutMax=[]  FilterDiffOutCoefMin=[]  FilterDiffOutCoefMax=[]  ReciprocalOutMin=[]  ReciprocalOutMax=[]  SumDenOutMin=[]  SumDenOutMax=[]  SumNumOutMin=[]  SumNumOutMax=[]  DivideOutMin=[]  DivideOutMax=[]  UdiffTsProdOutMin=[]  UdiffTsProdOutMax=[]  NTsProdOutMin=[]  NTsProdOutMax=[]  UintegralTsProdOutMin=[]  UintegralTsProdOutMax=[]  UngainTsProdOutMin=[]  UngainTsProdOutMax=[]  ClampingZeroOutDataTypeStr=Inherit: Inherit via back propagation  ClampingZeroOutMin=[]  ClampingZeroOutMax=[]  FilterDenConstantOutDataTypeStr=Inherit: Inherit via back propagation  FilterDenConstantOutMin=[]  FilterDenConstantOutMax=[]  PCopyOutDataTypeStr=Inherit: Inherit via back propagation  PCopyOutMin=[]  PCopyOutMax=[]  NCopyOutDataTypeStr=Inherit: Inherit via back propagation  NCopyOutMin=[]  NCopyOutMax=[]  IntegratorContinuousStateAttributes=''  IntegratorStateMustResolveToSignalObject=off  IntegratorRTWStateStorageClass=Auto  FilterContinuousStateAttributes=''  FilterStateMustResolveToSignalObject=off  FilterRTWStateStorageClass=Auto  ParallelPVariant=InternalParameters  IdealPVariant=Disabled  IVariant=InternalParameters  DVariant=InternalParameters  IntegratorVariant=Discrete  SatVariant=Disabled  AWVariant=Passthrough  PCopyVariant=Disabled  TRVariant=Disabled  FdbkBlocksVariant=Forward  IdealPFdbkVariant=Disabled  SatFdbkVariant=Disabled  DerivativeFilterVariant=ForwardEulerFilter  NVariant=InternalParameters  NCopyVariant=Disabled  FilterICVariant=InternalICsFilter  IntegratorICVariant=InternalICs  ExternalResetVariant=Disabled  TRSumVariant=Passthrough  SumFdbkVariant=Disabled  SumVariant=Sum_PID  TsampFilterVariant=InternalTs  TsampNgainVariant=Passthrough  TsampIntegralVariant=Disabled_SignalSpec  ExternalSaturationOutDataTypeStr=Inherit: Same as second input  DerivativeSourceVariant=ErrorSignal
  Altitude Controller : Subsystem
  Climb Rate SP Switch : Switch  Criteria=u2 > Threshold  SaturateOnIntegerOverflow=off  InputSameDT=off
  Climb Rate SP from Guidance : Subsystem  TreatAsAtomicUnit=on
  Compare To Constant : simulink/Logic and Bit Operations/Compare To Constant  relop===  const=uint8(1)  OutDataTypeStr=boolean
  Compare To Constant1 : simulink/Logic and Bit Operations/Compare To Constant  relop===  const=uint8(2)  OutDataTypeStr=boolean
  Pitch SP Controller : Subsystem
  Sum1 : Sum  Inputs=|+-
  Pitch SP : Outport
  Throttle : Outport  Port=2
  wires:
  Airspeed SP/1 -> Sum1/1
  Sum1/1 -> Airspeed Controller/1
  Airspeed/1 -> Sum1/2
  Airspeed Controller/1 -> Throttle/1
  Altitude SP/1 -> Altitude Controller/1(Alt SP)
  xyz/1 -> Altitude Controller/2(xyz)
  vxyz/1 -> Pitch SP Controller/2(vxyz)
  Pitch SP Controller/1(Pitch SP) -> Pitch SP/1
  Enable/1 -> Compare To Constant1/1, Compare To Constant/1
  Compare To Constant/1 -> Climb Rate SP Switch/2, Altitude Controller/Enable
  Compare To Constant1/1 -> Climb Rate SP from Guidance/Enable
  Altitude Controller/1(Climb Rate SP) -> Climb Rate SP Switch/1
  Climb Rate SP from Guidance/1(Out1) -> Climb Rate SP Switch/3
  Climb Rate SP Switch/1 -> Pitch SP Controller/1(Climb Rate SP)
  Climb Rate SP/1 -> Climb Rate SP from Guidance/1(Climb Rate SP)

== system Copy_of_VTOLTiltrotor/Flight Controller/Autopilot/Fixed Wing Controller/Fixed Wing Controller Tuning/Attitude Controller ==
  YPR SP : Inport
  ypr : Inport  Port=2
  Ang Rate : Inport  Port=3
  Airspeed : Inport  Port=4
  Enable : EnablePort  ShowOutputPort=on
  AER Switch : Switch  Criteria=u2 > Threshold  SaturateOnIntegerOverflow=off  InputSameDT=off
  Compare To Constant : simulink/Logic and Bit Operations/Compare To Constant  relop===  const=uint8(1)  OutDataTypeStr=boolean
  Compare To Constant1 : simulink/Logic and Bit Operations/Compare To Constant  relop===  const=uint8(2)  OutDataTypeStr=boolean
  Demux1 : Demux  Outputs=3
  Pitch Roll Controller : Subsystem
  Rudder Heading Controller : Subsystem
  AER : Outport
  wires:
  ypr/1 -> Rudder Heading Controller/2(YPR), Pitch Roll Controller/3(YPR)
  YPR SP/1 -> Demux1/1
  Enable/1 -> Compare To Constant1/1, Compare To Constant/1
  AER Switch/1 -> AER/1
  Compare To Constant/1 -> AER Switch/2, Pitch Roll Controller/Enable
  Pitch Roll Controller/1(AER) -> AER Switch/1
  Rudder Heading Controller/1(AER) -> AER Switch/3
  Demux1/1 -> Rudder Heading Controller/1(Yaw SP)
  Demux1/2 -> Pitch Roll Controller/1(Pitch SP)
  Demux1/3 -> Pitch Roll Controller/2(Roll SP)
  Ang Rate/1 -> Rudder Heading Controller/3(Ang Rate), Pitch Roll Controller/4(Ang Rate)
  Compare To Constant1/1 -> Rudder Heading Controller/Enable
  Airspeed/1 -> Pitch Roll Controller/5(Airspeed)

== system Copy_of_VTOLTiltrotor/Flight Controller/Autopilot/Fixed Wing Controller/Fixed Wing Controller Tuning/Lateral Guidance Logic ==
  note: S. Park, J. Deyst, and J. P. How, "A New Nonlinear Guidance Logic for Trajectory Tracking," Proceedings of the AIAA Guidance, Navigation and Control Conference, Aug 2004. AIAA-2004-4900.
  Course SP : Inport
  L1 Distance : Inport  Port=2
  course : Inport  Port=3
  gndspeed : Inport  Port=4
  Enable : EnablePort
  MATLAB Function : MATLAB Function  TreatAsAtomicUnit=on  SystemSampleTime=ControlSampleTime
  Terminator : Terminator
  Roll SP : Outport
  wires:
  Course SP/1 -> MATLAB Function/1(courseSP)
  course/1 -> MATLAB Function/2(course)
  MATLAB Function/2(rollSP) -> Roll SP/1
  MATLAB Function/1(lacc) -> Terminator/1
  gndspeed/1 -> MATLAB Function/3(groundSpeed)
  L1 Distance/1 -> MATLAB Function/4(L1)

== system Copy_of_VTOLTiltrotor/Flight Controller/Autopilot/Fixed Wing Controller/Fixed Wing Controller Tuning/Pitch, Airspeed SP from Controller ==
  Pitch SP In : Inport
  Airspeed SP : Inport  Port=2
  Airspeed : Inport  Port=3
  Enable : EnablePort
  Airspeed Controller : slpidlib/PID Controller  Controller=PID  Form=Parallel  TimeDomain=Discrete-time  UseExternalTs=off  SampleTime=ControlSampleTime  IntegratorMethod=Trapezoidal  FilterMethod=Forward Euler  ControllerParametersSource=internal  P=FWControlParams.P_AIRSPD  I=FWControlParams.I_AIRSPD  UseKiTs=off  D=FWControlParams.D_AIRSPD  UseExternalDerivativeSource=off  N=FWControlParams.N_AIRSPD  UseFilter=on  TunerSelectOption=Transfer Function Based (PID Tuner App)  InitialConditionSource=internal  InitialConditionForIntegrator=0  InitialConditionForFilter=0  DifferentiatorICPrevScaledInput=0  ExternalReset=none  TrackingMode=off  Kt=1  LimitOutput=off  SatLimitsSource=internal  UpperSaturationLimit=Inf  LowerSaturationLimit=0  LinearizeAsGain=on  AntiWindupMode=clamping  Kb=1  LimitIntegrator=off  UpperIntegratorSaturationLimit=inf  LowerIntegratorSaturationLimit=-inf  POutMin=[]  POutMax=[]  IOutMin=[]  IOutMax=[]  DOutMin=[]  DOutMax=[]  NOutMin=[]  NOutMax=[]  SumOutMin=[]  SumOutMax=[]  SaturationOutMin=[]  SaturationOutMax=[]  PParamMin=[]  PParamMax=[]  IParamMin=[]  IParamMax=[]  DParamMin=[]  DParamMax=[]  NParamMin=[]  NParamMax=[]  KbParamMin=[]  KbParamMax=[]  KtParamMin=[]  KtParamMax=[]  KbOutMin=[]  KbOutMax=[]  KtOutMin=[]  KtOutMax=[]  IntegratorOutMin=[]  IntegratorOutMax=[]  FilterOutMin=[]  FilterOutMax=[]  SumI1OutMin=[]  SumI1OutMax=[]  SumI2OutMin=[]  SumI2OutMax=[]  SumI3OutMin=[]  SumI3OutMax=[]  SumI4OutMin=[]  SumI4OutMax=[]  SumDOutMin=[]  SumDOutMax=[]  DifferentiatorOutMin=[]  DifferentiatorOutMax=[]  FilterDiffOutCoefMin=[]  FilterDiffOutCoefMax=[]  ReciprocalOutMin=[]  ReciprocalOutMax=[]  SumDenOutMin=[]  SumDenOutMax=[]  SumNumOutMin=[]  SumNumOutMax=[]  DivideOutMin=[]  DivideOutMax=[]  UdiffTsProdOutMin=[]  UdiffTsProdOutMax=[]  NTsProdOutMin=[]  NTsProdOutMax=[]  UintegralTsProdOutMin=[]  UintegralTsProdOutMax=[]  UngainTsProdOutMin=[]  UngainTsProdOutMax=[]  ClampingZeroOutDataTypeStr=Inherit: Inherit via back propagation  ClampingZeroOutMin=[]  ClampingZeroOutMax=[]  FilterDenConstantOutDataTypeStr=Inherit: Inherit via back propagation  FilterDenConstantOutMin=[]  FilterDenConstantOutMax=[]  PCopyOutDataTypeStr=Inherit: Inherit via back propagation  PCopyOutMin=[]  PCopyOutMax=[]  NCopyOutDataTypeStr=Inherit: Inherit via back propagation  NCopyOutMin=[]  NCopyOutMax=[]  IntegratorContinuousStateAttributes=''  IntegratorStateMustResolveToSignalObject=off  IntegratorRTWStateStorageClass=Auto  FilterContinuousStateAttributes=''  FilterStateMustResolveToSignalObject=off  FilterRTWStateStorageClass=Auto  ParallelPVariant=InternalParameters  IdealPVariant=Disabled  IVariant=InternalParameters  DVariant=InternalParameters  IntegratorVariant=Discrete  SatVariant=Disabled  AWVariant=Passthrough  PCopyVariant=Disabled  TRVariant=Disabled  FdbkBlocksVariant=Forward  IdealPFdbkVariant=Disabled  SatFdbkVariant=Disabled  DerivativeFilterVariant=ForwardEulerFilter  NVariant=InternalParameters  NCopyVariant=Disabled  FilterICVariant=InternalICsFilter  IntegratorICVariant=InternalICs  ExternalResetVariant=Disabled  TRSumVariant=Passthrough  SumFdbkVariant=Disabled  SumVariant=Sum_PID  TsampFilterVariant=InternalTs  TsampNgainVariant=Passthrough  TsampIntegralVariant=Disabled_SignalSpec  ExternalSaturationOutDataTypeStr=Inherit: Same as second input  DerivativeSourceVariant=ErrorSignal
  IC : InitialCondition  Value=0
  Sum1 : Sum  Inputs=|+-
  Pitch SP : Outport
  Throttle : Outport  Port=2
  wires:
  IC/1 -> Pitch SP/1
  Pitch SP In/1 -> IC/1
  Airspeed SP/1 -> Sum1/1
  Sum1/1 -> Airspeed Controller/1
  Airspeed/1 -> Sum1/2
  Airspeed Controller/1 -> Throttle/1

== system Copy_of_VTOLTiltrotor/Flight Controller/Autopilot/Fixed Wing Controller/Fixed Wing Controller Tuning/Roll SP from Path Manager ==
  In1 : Inport
  Enable : EnablePort
  IC : InitialCondition  Value=0
  Out1 : Outport
  wires:
  In1/1 -> IC/1
  IC/1 -> Out1/1

== system Copy_of_VTOLTiltrotor/Flight Controller/Autopilot/Fixed Wing Controller/Fixed Wing Controller Tuning/Subsystem2 ==
  Euler : Inport
  pqr : Inport  Port=2
  Demux : Demux  Outputs=3
  Display : Display
  MATLAB Function : MATLAB Function  TreatAsAtomicUnit=on
  Matrix Multiply : Product  Multiplication=Matrix(*)
  Terminator : Terminator
  Euler Rate : Outport
  wires:
  Demux/1 -> MATLAB Function/1(phi)
  Demux/2 -> MATLAB Function/2(theta)
  MATLAB Function/1(y) -> Matrix Multiply/1
  pqr/1 -> Matrix Multiply/2
  Euler/1 -> Demux/1
  Demux/3 -> Terminator/1
  Matrix Multiply/1 -> Display/1, Euler Rate/1

== system Copy_of_VTOLTiltrotor/Flight Controller/Autopilot/Multicopter Controller/Altitude Control/Triggered Subsystem ==
  AltHold : Inport
  Trigger : TriggerPort  VariantControl=(inherit)
  Reference : Outport
  wires:
  AltHold/1 -> Reference/1
